simulink model "LinearActuator"  (R2018a)
settings: Solver=ode45  StartTime=0.0  StopTime=10.0  MaxStep=0.1  RelTol=1e-3  EnableMultiTasking=on
undefined symbols (not defined in the file): Ta
settings Model: DataDictionary=system_model.sldd  FPTRunName=Active  ModifiedByFormat=The MathWorks Inc.  Creator=The MathWorks, Inc.  LastModifiedBy=The MathWorks Inc.
settings DataIOCC: LimitDataPoints=on  SaveFormat=Array  SaveOutput=off  SignalLogging=off  SaveTime=off  SignalLoggingName=LinearActuator
settings OptimizationCC: ExpressionDepthLimit=2147483647  InitFltsAndDblsToZero=on  LifeSpan=inf
settings DebuggingCC: SaveWithParameterizedLinksMsg=none  UnderspecifiedInitializationDetection=Classic  MergeDetectMultiDrivingBlocksExec=none  SignalResolutionControl=TryResolveAllWithWarning  SolverPrmCheckMsg=warning  MultiTaskDSMMsg=warning  MultiTaskCondExecSysMsg=none  FcnCallInpInsideContextMsg=warning  AllowSymbolicDim=off  StateNameClashWarn=warning  SFUnexpectedBacktrackingDiag=warning  SFNoUnconditionalDefaultTransitionDiag=warning  SFExecutionAtInitializationDiag=none
settings HardwareCC: ProdBitPerPointer=32  ProdLargestAtomicFloat=None  ProdIntDivRoundTo=Undefined  ProdEndianess=Unspecified  ProdWordSize=32  ProdHWDeviceType=32-bit Generic
settings ModelReferenceCC: ModelReferenceMinAlgLoopOccurrences=on  PropagateSignalLabelsOutOfModel=off
settings CodeAppCC: StateflowObjectComments=on
settings GRTTargetCC: TargetFcnLib=ansi_tfl_tmw.mat  TargetLangStandard=C89/C90 (ANSI)  GeneratePreprocessorConditionals=Disable all  CombineOutputUpdateFcns=off  GRTInterface=on
settings ConfigComp: CovMetricSettings=dw  CovHtmlReporting=on  CovSaveCumulativeToWorkspaceVar=on  CovSaveSingleToWorkspaceVar=on  CovExternalEMLEnable=off  CovSFcnEnable=off

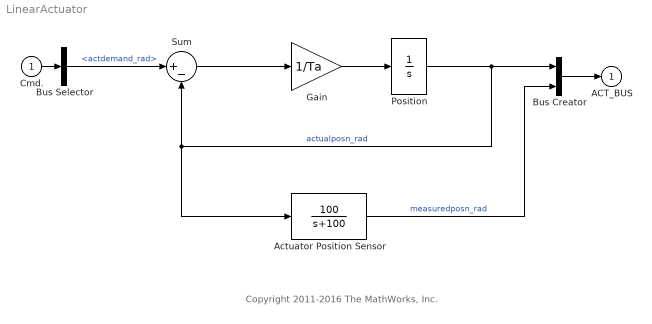
== system LinearActuator ==
  note: Copyright 2011-2016 The MathWorks, Inc.
  Cmd. : Inport  OutDataTypeStr=Bus: CONTROL_BUS
  Actuator Position Sensor : TransferFcn  Numerator=[100]  Denominator=[1 100]
  Bus Creator : BusCreator  Inputs=2  OutDataTypeStr=Bus: ACT_BUS
  Bus Selector : BusSelector  OutputSignals=actdemand_rad
  Gain : Gain  Gain=1/Ta  SaturateOnIntegerOverflow=on  OutDataTypeStr=Inherit: Same as input  ParamDataTypeStr=Inherit: Same as input
  Position : Integrator  UpperSaturationLimit=pi*45/180  LowerSaturationLimit=-pi*45/180
  Sum : Sum  Inputs=|+-  SaturateOnIntegerOverflow=on  InputSameDT=on  OutDataTypeStr=Inherit: Same as first input
  ACT_BUS : Outport  OutDataTypeStr=Bus: ACT_BUS  InitialOutput=0  BusOutputAsStruct=on
  wires:
  Actuator Position Sensor/1 -> Bus Creator/2  "measuredposn_rad"
  Position/1 -> Bus Creator/1, Actuator Position Sensor/1, Sum/2  "actualposn_rad"
  Gain/1 -> Position/1
  Sum/1 -> Gain/1
  Cmd./1 -> Bus Selector/1
  Bus Selector/1 -> Sum/1  "<actdemand_rad>"
  Bus Creator/1 -> ACT_BUS/1
